simulink model "gm_lorenz_model"  (R2018a)
settings: Solver=FixedStepAuto  StartTime=0.0  StopTime=inf  RelTol=1e-3  EnableMultiTasking=on
libraries: simulink_extras x1
settings Model: Creator=labuser  LastModifiedBy=labuser
settings SolverCC: PositivePriorityOrder=on
settings OptimizationCC: BlockReduction=off  ConditionallyExecuteInputs=off  DefaultParameterBehavior=Inlined  EnhancedBackFolding=on  PassReuseOutputArgsThreshold=0  MaxStackSize=64  OptimizeBlockOrder=speed  DifferentSizesBufferReuse=on  OptimizationCustomize=off
settings DebuggingCC: AlgebraicLoopMsg=error  InheritedTsInSrcMsg=none  ParameterTunabilityLossMsg=error
settings HardwareCC: ProdBitPerPointer=32  ProdBitPerSizeT=32  ProdBitPerPtrDiffT=32  ProdLargestAtomicFloat=None  ProdIntDivRoundTo=Undefined  ProdEndianess=Unspecified  ProdWordSize=32  ProdHWDeviceType=ASIC/FPGA->ASIC/FPGA  TargetBitPerPointer=64  TargetBitPerSizeT=64  TargetBitPerPtrDiffT=64  TargetLongLongMode=on  TargetIntDivRoundTo=Zero  TargetEndianess=LittleEndian  TargetWordSize=64  TargetHWDeviceType=Custom Processor->MATLAB Host Computer  ProdEqTarget=off
settings SFSimCC: MATLABDynamicMemAlloc=off
settings RTWCC: Description=Generic Real-Time Target  GenerateReport=on  Toolchain=ARM Development Studio Altera Edition (DS-5 AE)  LaunchReport=on
settings CodeAppCC: ForceParamTrailComments=on  OperatorAnnotations=on
settings GRTTargetCC: TargetLangStandard=C89/C90 (ANSI)

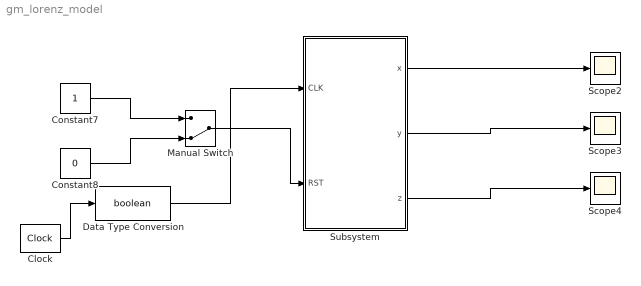
== system gm_lorenz_model ==
  Clock : simulink_extras/Flip Flops/Clock  period=1
  Constant7 : Constant  OutDataTypeStr=boolean  SampleTime=-1
  Constant8 : Constant  Value=0  OutDataTypeStr=boolean  SampleTime=-1
  Data Type Conversion : DataTypeConversion  OutDataTypeStr=boolean
  Manual Switch : ManualSwitch  CurrentSetting=0
  Scope2 : Scope
  Scope3 : Scope
  Scope4 : Scope
  Subsystem : Subsystem  TreatAsAtomicUnit=on
  wires:
  Data Type Conversion/1 -> Subsystem/1(CLK)
  Clock/1 -> Data Type Conversion/1
  Manual Switch/1 -> Subsystem/2(RST)
  Constant8/1 -> Manual Switch/2
  Constant7/1 -> Manual Switch/1
  Subsystem/2(y) -> Scope3/1
  Subsystem/3(z) -> Scope4/1
  Subsystem/1(x) -> Scope2/1

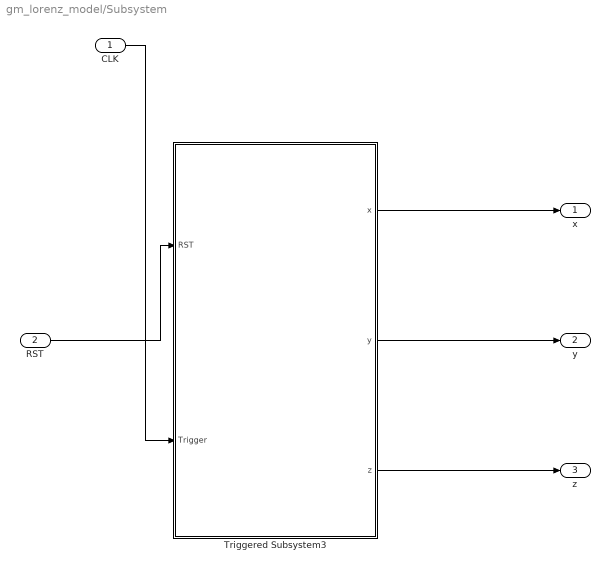
== system gm_lorenz_model/Subsystem ==
  CLK : Inport  OutDataTypeStr=boolean  PortDimensions=1  SampleTime=0.5
  RST : Inport  Port=2  OutDataTypeStr=boolean  PortDimensions=1  SampleTime=0.5
  Triggered Subsystem3 : Subsystem
  x : Outport  OutDataTypeStr=fixdt(1,27,20)
  y : Outport  Port=2  OutDataTypeStr=fixdt(1,27,20)
  z : Outport  Port=3  OutDataTypeStr=fixdt(1,27,20)
  wires:
  CLK/1 -> Triggered Subsystem3/2(Trigger)
  RST/1 -> Triggered Subsystem3/1(RST)
  Triggered Subsystem3/1(x) -> x/1
  Triggered Subsystem3/2(y) -> y/1
  Triggered Subsystem3/3(z) -> z/1

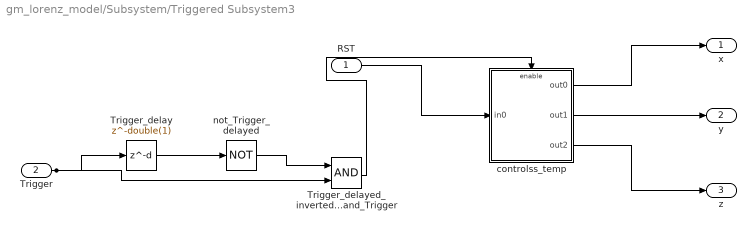
== system gm_lorenz_model/Subsystem/Triggered Subsystem3 ==
  RST : Inport  OutDataTypeStr=boolean  PortDimensions=1  SampleTime=0.5
  Trigger : Inport  Port=2  OutDataTypeStr=boolean  SampleTime=0.5
  Trigger_delay : Delay  DelayLength=double(1)  InitialCondition=1  InputProcessing=Inherited
  Trigger_delayed_inverted_and_Trigger : Logic  AllPortsSameDT=off  OutDataTypeStr=boolean  SampleTime=0.5
  controlss_temp : Subsystem
  not_Trigger_delayed : Logic  Operator=NOT  Inputs=1  AllPortsSameDT=off  OutDataTypeStr=boolean  SampleTime=0.5
  x : Outport  OutDataTypeStr=fixdt(1,27,20)  InitialOutput=0
  y : Outport  Port=2  OutDataTypeStr=fixdt(1,27,20)  InitialOutput=0
  z : Outport  Port=3  OutDataTypeStr=fixdt(1,27,20)  InitialOutput=0
  wires:
  Trigger/1 -> Trigger_delayed_inverted_and_Trigger/2, Trigger_delay/1
  RST/1 -> controlss_temp/1(in0)
  controlss_temp/1(out0) -> x/1
  controlss_temp/2(out1) -> y/1
  controlss_temp/3(out2) -> z/1
  Trigger_delay/1 -> not_Trigger_delayed/1
  not_Trigger_delayed/1 -> Trigger_delayed_inverted_and_Trigger/1
  Trigger_delayed_inverted_and_Trigger/1 -> controlss_temp/Enable

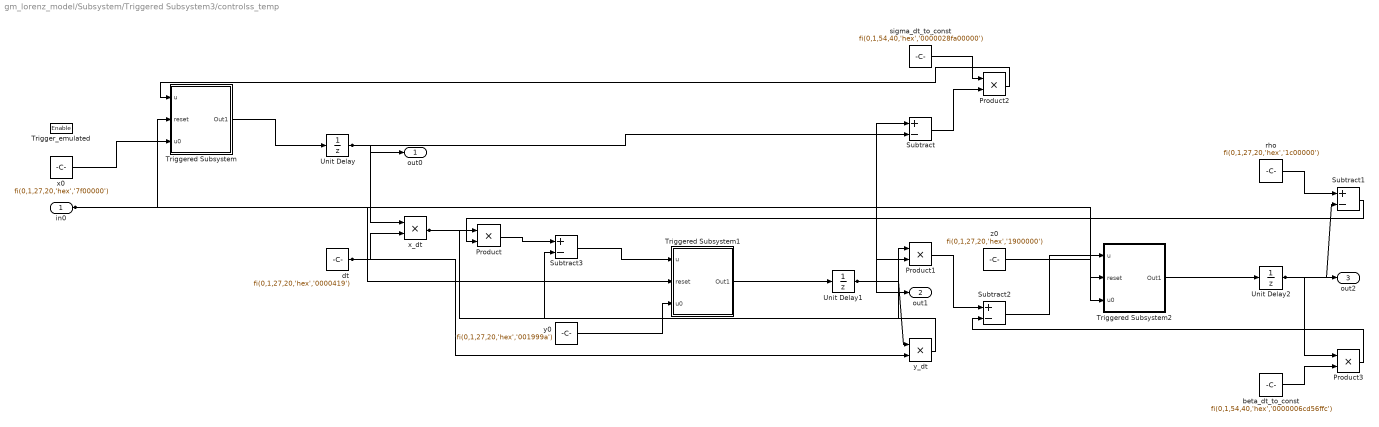
== system gm_lorenz_model/Subsystem/Triggered Subsystem3/controlss_temp ==
  in0 : Inport  OutDataTypeStr=boolean  SampleTime=0.5
  Trigger_emulated : EnablePort  OutDataTypeStr=boolean
  Product{,1..3} (4 alike) : Product  Inputs=**  OutDataTypeStr=fixdt(1, 27, 20)  SampleTime=0.5
  Subtract{,1..3} (4 alike) : Sum  Inputs=+-  AccumDataTypeStr=fixdt(1, 27, 20)  OutDataTypeStr=fixdt(1, 27, 20)  SampleTime=0.5
  Triggered Subsystem : Subsystem
  Triggered Subsystem1 : Subsystem
  Triggered Subsystem2 : Subsystem
  Unit Delay : UnitDelay  InitialCondition=fi(0,1,27,20,'hex','0000000')  SampleTime=0.5
  Unit Delay1 : UnitDelay  InitialCondition=fi(0,1,27,20,'hex','0000000')  SampleTime=0.5
  Unit Delay2 : UnitDelay  InitialCondition=fi(0,1,27,20,'hex','0000000')  SampleTime=0.5
  beta_dt_to_const : Constant  Value=fi(0,1,54,40,'hex','0000006cd56ffc')  OutDataTypeStr=fixdt(1, 27, 20)  SampleTime=-1
  "dt " : Constant  Value=fi(0,1,27,20,'hex','0000419')  OutDataTypeStr=fixdt(1, 27, 20)  SampleTime=-1
  rho : Constant  Value=fi(0,1,27,20,'hex','1c00000')  OutDataTypeStr=fixdt(1, 27, 20)  SampleTime=-1
  sigma_dt_to_const : Constant  Value=fi(0,1,54,40,'hex','0000028fa00000')  OutDataTypeStr=fixdt(1, 27, 20)  SampleTime=-1
  x0 : Constant  Value=fi(0,1,27,20,'hex','7f00000')  OutDataTypeStr=fixdt(1, 27, 20)  SampleTime=-1
  x_dt : Product  Inputs=**  OutDataTypeStr=fixdt(1, 27, 20)  SampleTime=0.5
  y0 : Constant  Value=fi(0,1,27,20,'hex','001999a')  OutDataTypeStr=fixdt(1, 27, 20)  SampleTime=-1
  y_dt : Product  Inputs=**  OutDataTypeStr=fixdt(1, 27, 20)  SampleTime=0.5
  z0 : Constant  Value=fi(0,1,27,20,'hex','1900000')  OutDataTypeStr=fixdt(1, 27, 20)  SampleTime=-1
  out0 : Outport  OutDataTypeStr=fixdt(1, 27, 20)  InitialOutput=0
  out1 : Outport  Port=2  OutDataTypeStr=fixdt(1, 27, 20)  InitialOutput=0
  out2 : Outport  Port=3  OutDataTypeStr=fixdt(1, 27, 20)  InitialOutput=0
  wires:
  Product/1 -> Subtract3/1
  Product1/1 -> Subtract2/1
  Product2/1 -> Triggered Subsystem/1(u)
  Product3/1 -> Subtract2/2
  Subtract/1 -> Product2/2
  Subtract1/1 -> Product/2
  Subtract2/1 -> Triggered Subsystem2/1(u)
  Subtract3/1 -> Triggered Subsystem1/1(u)
  Triggered Subsystem/1(Out1) -> Unit Delay/1
  Triggered Subsystem1/1(Out1) -> Unit Delay1/1
  Triggered Subsystem2/1(Out1) -> Unit Delay2/1
  beta_dt_to_const/1 -> Product3/2
  sigma_dt_to_const/1 -> Product2/1
  x_dt/1 -> Product1/1, Product/1
  y_dt/1 -> Subtract3/2
  Unit Delay/1 -> x_dt/1, Subtract/2, out0/1
  Unit Delay1/1 -> y_dt/1, Subtract/1, Product1/2, out1/1
  Unit Delay2/1 -> Subtract1/2, Product3/1, out2/1
  "dt "/1 -> y_dt/2, x_dt/2
  rho/1 -> Subtract1/1
  x0/1 -> Triggered Subsystem/3(u0)
  y0/1 -> Triggered Subsystem1/3(u0)
  z0/1 -> Triggered Subsystem2/3(u0)
  in0/1 -> Triggered Subsystem/2(reset), Triggered Subsystem1/2(reset), Triggered Subsystem2/2(reset)

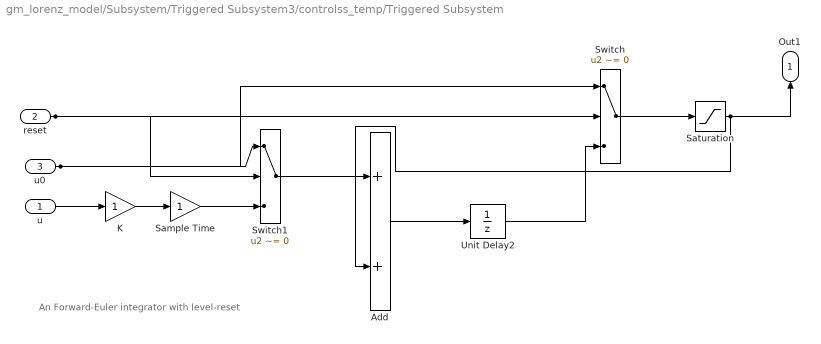
== system gm_lorenz_model/Subsystem/Triggered Subsystem3/controlss_temp/Triggered Subsystem ==
  note: An Forward-Euler integrator with level-reset
  u : Inport  PortDimensions=1  SampleTime=0.5
  reset : Inport  Port=2  PortDimensions=1  SampleTime=0.5
  u0 : Inport  Port=3  PortDimensions=1  SampleTime=0.5
  Add : Sum
  K : Gain  OutDataTypeStr=Inherit: Same as input
  Sample Time : Gain  OutDataTypeStr=Inherit: Same as input
  Saturation : Saturate  UpperLimit=63  LowerLimit=-63
  Switch : Switch  Criteria=u2 ~= 0  OutDataTypeStr=Inherit: Inherit via back propagation
  Switch1 : Switch  Criteria=u2 ~= 0  OutDataTypeStr=Inherit: Inherit via back propagation
  Unit Delay2 : UnitDelay  SampleTime=-1
  Out1 : Outport  InitialOutput=0
  wires:
  u/1 -> K/1
  reset/1 -> Switch1/2, Switch/2
  u0/1 -> Switch1/1, Switch/1
  Add/1 -> Unit Delay2/1
  K/1 -> Sample Time/1
  Sample Time/1 -> Switch1/3
  Saturation/1 -> Add/2, Out1/1
  Switch/1 -> Saturation/1
  Switch1/1 -> Add/1
  Unit Delay2/1 -> Switch/3

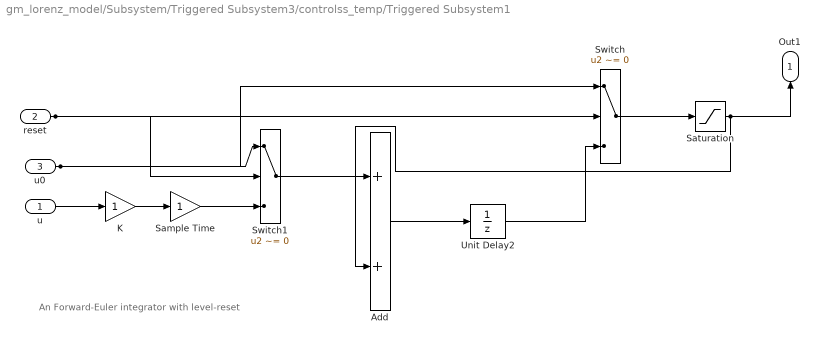
== system gm_lorenz_model/Subsystem/Triggered Subsystem3/controlss_temp/Triggered Subsystem1 ==
  note: An Forward-Euler integrator with level-reset
  u : Inport  PortDimensions=1  SampleTime=0.5
  reset : Inport  Port=2  PortDimensions=1  SampleTime=0.5
  u0 : Inport  Port=3  PortDimensions=1  SampleTime=0.5
  Add : Sum
  K : Gain  OutDataTypeStr=Inherit: Same as input
  Sample Time : Gain  OutDataTypeStr=Inherit: Same as input
  Saturation : Saturate  UpperLimit=63  LowerLimit=-63
  Switch : Switch  Criteria=u2 ~= 0  OutDataTypeStr=Inherit: Inherit via back propagation
  Switch1 : Switch  Criteria=u2 ~= 0  OutDataTypeStr=Inherit: Inherit via back propagation
  Unit Delay2 : UnitDelay  SampleTime=-1
  Out1 : Outport  InitialOutput=0
  wires:
  Unit Delay2/1 -> Switch/3
  Switch1/1 -> Add/1
  Switch/1 -> Saturation/1
  Saturation/1 -> Out1/1, Add/2
  Sample Time/1 -> Switch1/3
  K/1 -> Sample Time/1
  Add/1 -> Unit Delay2/1
  u0/1 -> Switch/1, Switch1/1
  reset/1 -> Switch/2, Switch1/2
  u/1 -> K/1

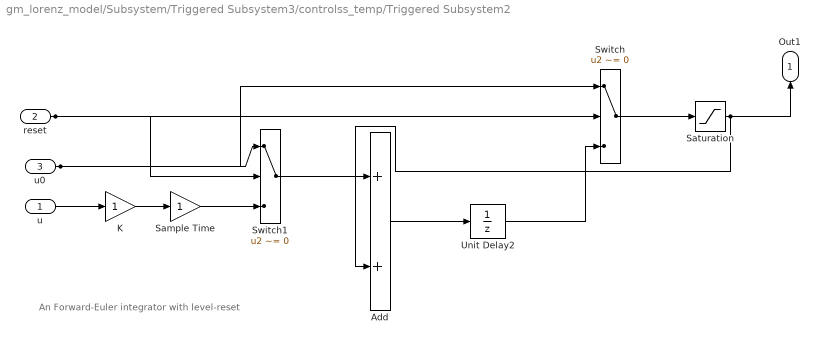
== system gm_lorenz_model/Subsystem/Triggered Subsystem3/controlss_temp/Triggered Subsystem2 ==
  note: An Forward-Euler integrator with level-reset
  u : Inport  PortDimensions=1  SampleTime=0.5
  reset : Inport  Port=2  PortDimensions=1  SampleTime=0.5
  u0 : Inport  Port=3  PortDimensions=1  SampleTime=0.5
  Add : Sum
  K : Gain  OutDataTypeStr=Inherit: Same as input
  Sample Time : Gain  OutDataTypeStr=Inherit: Same as input
  Saturation : Saturate  UpperLimit=63  LowerLimit=-63
  Switch : Switch  Criteria=u2 ~= 0  OutDataTypeStr=Inherit: Inherit via back propagation
  Switch1 : Switch  Criteria=u2 ~= 0  OutDataTypeStr=Inherit: Inherit via back propagation
  Unit Delay2 : UnitDelay  SampleTime=-1
  Out1 : Outport  InitialOutput=0
  wires:
  Unit Delay2/1 -> Switch/3
  Switch1/1 -> Add/1
  Switch/1 -> Saturation/1
  Saturation/1 -> Out1/1, Add/2
  Sample Time/1 -> Switch1/3
  K/1 -> Sample Time/1
  Add/1 -> Unit Delay2/1
  u0/1 -> Switch/1, Switch1/1
  reset/1 -> Switch/2, Switch1/2
  u/1 -> K/1
